simulink model "rls_filt_direct_form_simulink"  (R2016a)
settings: Solver=VariableStepAuto  StartTime=0.0  StopTime=inf  RelTol=1e-3
libraries: dspsrcs4 x2, dsparch4 x1
settings Model: Creator=User  LastModifiedBy=User

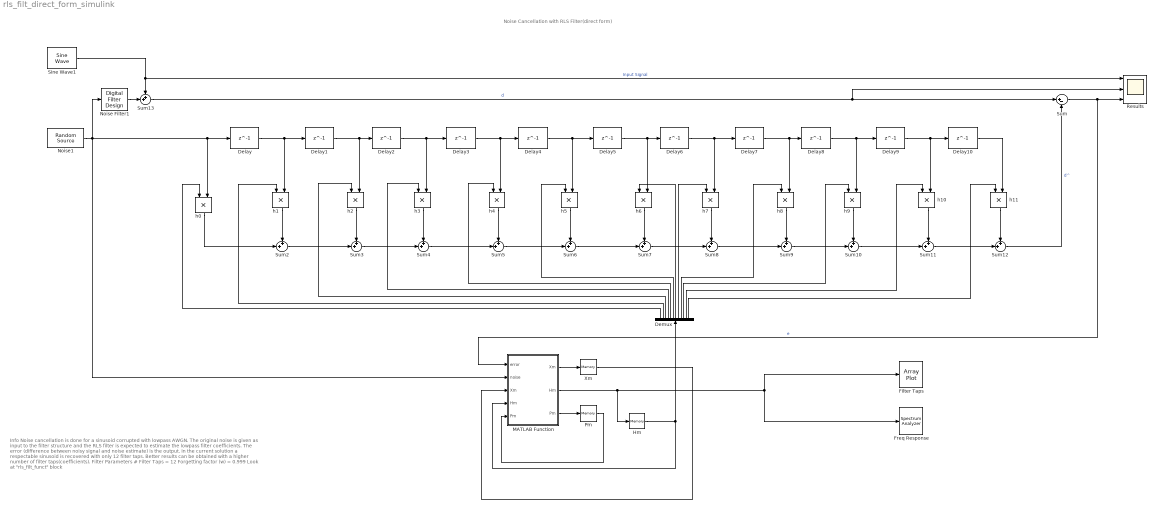
== system rls_filt_direct_form_simulink ==
  note: Info
      | Noise cancellation is done for a sinusoid corrupted with lowpass AWGN.
      | The original noise is given as input to the filter structure and the RLS filter is
      | expected to estimate the lowpass filter coefficients. The error (difference
      | between noisy signal and noise estimate) is the output. In the current solution
      | a respectable sinusoid is recovered with only 12 filter taps. Better results can
      | be obtained with a higher number of filter taps(coefficients).
      |
      | Filter Parameters
      | # Filter Taps = 12
      | Forgetting factor (w) = 0.999
      | Look at "rls_filt_funct" block
  note: Noise Cancellation with RLS Filter(direct form)
  Delay{,1..10} (11 alike) : Delay  DelayLength=1  InputProcessing=Columns as channels (frame based)
  Demux : Demux  Outputs=12
  Filter Taps : ArrayPlot
  Freq Response : SpectrumAnalyzer
  Hm : Memory  X0=zeros(12, 1)  InheritSampleTime=on
  MATLAB Function : MATLAB Function  TreatAsAtomicUnit=on
  Noise Filter1 : dsparch4/Digital Filter Design  mwdsp_browser_bugfix_var=off
  Noise1 : dspsrcs4/Random Source  SrcType=Gaussian  NormMethod=Ziggurat  CltLength=12  MinVal=0  MaxVal=1  MeanVal=0  VarVal=1  RepMode=Specify seed  rawSeed=[23341]  IsInherit=off  SampMode=Discrete  SampTime=1  SampFrame=1  DataType=Double  OutComplex=Real  OutputFrames=on
  Pm : Memory  X0=0.01*eye(12)  InheritSampleTime=on
  Results : Scope  NumInputPorts=3
  Sine Wave1 : dspsrcs4/Sine Wave  Amplitude=1  Frequency=0.055  Phase=0  SampleMode=Discrete  OutComplex=Real  CompMethod=Trigonometric fcn  TableSize=Speed  SampleTime=1  SamplesPerFrame=1  ResetState=Restart at time zero  OutputFrames=on  dataType=double  wordLen=16  udDataType=sfix(16)  fracBitsMode=User-defined  numFracBits=14  OutDataTypeStr=double  LastOutDataTypeStr=double
  Sum : Sum  Inputs=|+-
  Sum{2..12} (11 alike) : Sum  Inputs=++|
  Sum13 : Sum  Inputs=++|  SaturateOnIntegerOverflow=on  InputSameDT=on  OutDataTypeStr=Inherit: Same as first input
  Xm : Memory  X0=zeros(12, 1)  InheritSampleTime=on
  h{0..11} (12 alike) : Product
  wires:
  MATLAB Function/2(Hm) -> Freq Response/1, Filter Taps/1, Hm/1
  MATLAB Function/1(Xm) -> Xm/1
  Xm/1 -> MATLAB Function/3("Xm ")
  Hm/1 -> MATLAB Function/4("Hm "), Demux/1
  MATLAB Function/3(Pm) -> Pm/1
  Pm/1 -> MATLAB Function/5("Pm ")
  h1/1 -> Sum2/1
  Delay/1 -> h1/2, Delay1/1
  Sum2/1 -> Sum3/2
  Sum3/1 -> Sum4/2
  Sum4/1 -> Sum5/2
  Sum5/1 -> Sum6/2
  Sum6/1 -> Sum7/2
  h2/1 -> Sum3/1
  Delay1/1 -> h2/2, Delay2/1
  h3/1 -> Sum4/1
  Delay2/1 -> h3/2, Delay3/1
  h4/1 -> Sum5/1
  Delay3/1 -> h4/2, Delay4/1
  h5/1 -> Sum6/1
  Delay4/1 -> h5/2, Delay5/1
  h6/1 -> Sum7/1
  Delay5/1 -> Delay6/1, h6/2
  h7/1 -> Sum8/1
  Delay6/1 -> h7/2, Delay7/1
  Sum8/1 -> Sum9/2
  Sum9/1 -> Sum10/2
  Sum10/1 -> Sum11/2
  Sum11/1 -> Sum12/2
  h8/1 -> Sum9/1
  Delay7/1 -> h8/2, Delay8/1
  h9/1 -> Sum10/1
  Delay8/1 -> h9/2, Delay9/1
  h10/1 -> Sum11/1
  Delay9/1 -> h10/2, Delay10/1
  h11/1 -> Sum12/1
  Delay10/1 -> h11/2
  Sum7/1 -> Sum8/2
  h0/1 -> Sum2/2
  Sine Wave1/1 -> Results/1, Sum13/1  "Input Signal"
  Noise1/1 -> MATLAB Function/2(noise), Noise Filter1/1, h0/2, Delay/1
  Sum13/1 -> Results/2, Sum/1  "d"
  Sum12/1 -> Sum/2  "d^"
  Sum/1 -> MATLAB Function/1(error), Results/3  "e"
  Demux/1 -> h0/1
  Demux/2 -> h1/1
  Demux/3 -> h2/1
  Demux/4 -> h3/1
  Demux/5 -> h4/1
  Demux/6 -> h5/1
  Demux/7 -> h6/1
  Demux/8 -> h7/1
  Demux/9 -> h8/1
  Demux/10 -> h9/1
  Demux/11 -> h10/1
  Demux/12 -> h11/1
  Noise Filter1/1 -> Sum13/2

== matlab function rls_filt_direct_form_simulink/MATLAB Function ==
  data: error input; Xm output; noise input; Hm output; Xm input; Hm input; Pm input; Pm output
function [Xm, Hm, Pm] = rls_filt_funct(error, noise, Xm, Hm, Pm)
%
% Function for RLS filter coeffients computation
%
% error: difference between signal and estimated noise at time n
% noise: original noise at time n
% Xm(M, 1) : noise vector (window)
% Hm(M, 1) : filter coefficients
% Pm(M, M) : inverse correction matrix
% 

M = 12;
w = 0.999;

Xm = [noise; Xm(1:M-1)]; % calculate Xm(n) from Xm(n-1)          

% kalman gain vector
Km = (Pm*Xm)/(w + Xm'*Pm*Xm);

% update inverse correlation matrix
Pm = (1/w)*(Pm - Km*Xm'*Pm);

% update filter coefficients
Hm = Hm + Km*error;
